simulink model "circuit2"  (Simulink 5.0)
settings: Solver=ode23tb  StartTime=0.0  StopTime=0.02  RelTol=1e-3
libraries: powerlib2 x15
settings Model: LastModifiedBy=Администратор

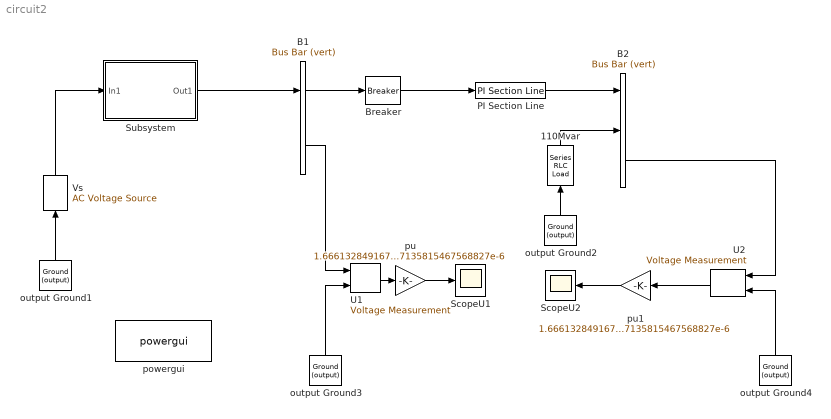
== system circuit2 ==
  110Mvar : powerlib2/Elements/Series RLC Load  Tag=PoWeRsYsTeMbLoCk  Orientation=up  a=424.4e3  b=60  c=0.366666666667e6  d=110e6  e=0  mesure=None  PSBOutputType=1
  B1 : powerlib2/Connectors/Bus Bar (vert)  Tag=PoWeRsYsTeMbLoCk  entrees=2  sorties=2  PSBOutputType=11111111111111111111111111111111111111111111111111111111111111111111111111111111111111111
  B2 : powerlib2/Connectors/Bus Bar (vert)  Tag=PoWeRsYsTeMbLoCk  entrees=3  sorties=2  PSBOutputType=11111111111111111111111111111111111111111111111111111111111111111111111111111111111111111
  Breaker : powerlib2/Elements/Breaker  Tag=PoWeRsYsTeMbLoCk  a=0.001  c=0  rs=inf  cs=0  times=[(1/60)/4]  Ts=0  comext=off  mesure=None  PSBOutputType=1
  PI Section Line : powerlib2/Elements/PI Section Line  Tag=PoWeRsYsTeMbLoCk  f=60  a=0.011  b=0.8674e-03  c=13.41e-09  d=300  e=10  mesure=None  PSBOutputType=1
  ScopeU1 : Scope
      settings: YMin=-1.25  YMax=1.25
  ScopeU2 : Scope
      settings: TimeRange=0.02  YMin=-6.97024  YMax=-2.97024  SaveName=U2  DataFormat=Array
  Subsystem : Subsystem
      mask Display: disp ('Equivalent\nCircuit')
  U1 : powerlib2/Measurements/Voltage Measurement  Tag=PoWeRsYsTeMmEaSuReMeNt  PhasorSimulation=off  OutputType=Magnitude  PSBOutputType=0  PSBequivalent=0
  U2 : powerlib2/Measurements/Voltage Measurement  Tag=PoWeRsYsTeMmEaSuReMeNt  Orientation=left  PhasorSimulation=off  OutputType=Magnitude  PSBOutputType=0  PSBequivalent=1
  Vs : powerlib2/Electrical Sources/AC Voltage Source  Tag=PoWeRsYsTeMbLoCk  Description=source block  Orientation=up  A=600192.2358711415387114366945546  P=0  F=60  stime=0  mesure=None  PSBOutputType=1
  output Ground{1..4} (4 alike) : powerlib2/Connectors/Ground (output)  Tag=PoWeRsYsTeMbLoCk  Orientation=up  PSBOutputType=1
  powergui : powerlib2/powergui  Priority=2  Frange=[0:2:1500]  Ylog=on  Xlog=off  save=on  variable=ZData  ZoomFFT=on  StartTime=0.0  cycles=1  DisplayStyle=1  fundamental=60  FreqAxis=off  MaxFrequency=1000  frequencyindice=1  frequencyindicesteady=1  RmsSteady=1  display=off  Ts=0  methode=off  frequency=60  echomessages=off
  pu : Gain  Gain=1.66613284916717135815467568827e-6  SaturateOnIntegerOverflow=on
  pu1 : Gain  Orientation=left  Gain=1.66613284916717135815467568827e-6  SaturateOnIntegerOverflow=on
  wires:
  Vs/1 -> Subsystem/1(In1)
  output Ground1/1 -> Vs/1
  Subsystem/1(Out1) -> B1/1
  B1/1 -> Breaker/1
  PI Section Line/1 -> B2/1
  110Mvar/1 -> B2/2
  output Ground2/1 -> 110Mvar/1
  B1/2 -> U1/1
  output Ground3/1 -> U1/2
  U1/1 -> pu/1
  pu/1 -> ScopeU1/1
  U2/1 -> pu1/1
  pu1/1 -> ScopeU2/1
  B2/2 -> U2/1
  output Ground4/1 -> U2/2
  Breaker/1 -> PI Section Line/1

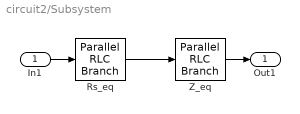
== system circuit2/Subsystem ==
  In1 : Inport
  Rs_eq : powerlib2/Elements/Parallel RLC Branch  Tag=PoWeRsYsTeMbLoCk  a=2  b=inf  c=0  mesure=None  PSBOutputType=1
  Z_eq : powerlib2/Elements/Parallel RLC Branch  Tag=PoWeRsYsTeMbLoCk  a=180.1  b=26.525e-03  c=117.84e-06  mesure=None  PSBOutputType=1
  Out1 : Outport
  wires:
  Rs_eq/1 -> Z_eq/1
  In1/1 -> Rs_eq/1
  Z_eq/1 -> Out1/1
